simulink model "CAN_new"  (R2013b)
settings: Solver=FixedStepDiscrete  StartTime=0.0  StopTime=Inf  FixedStep=0.001  RelTol=1e-3
PostLoadFcn:
  | , if any(exist('dsrtsu_mdlpostloadfcn', 'file') == [2, 3, 6]), try dsrtsu_mdlpostloadfcn('Execute', bdroot); catch fprintf('Error in PostLoadFcn (dsrtsu_mdlpostloadfcn) for model "%s":\n %s\n', bdroot, lasterr); end, end,
undefined symbols (not defined in the file or in its folder): rticanmm_blockfcn, rticanmm_initfcn
libraries: rtimmsu_dsrtlib x4
(part 1 of 2)
settings Model: DSRTSU_INTERNAL_RTI_VER=440  DSRTSU_INTERNAL_RTI_TYPE=rti1401  RTICANMMDATA=struct('GeneralSetupData',struct('modelroot','C:\Users\Sebastian\Documents\GitHub\MA_Active_Steering_Dolly\DBC_Files','generalsettings',struct('filesettings',struct('destfolder',struct('Name','RTICANMM_FILES','Check',1),'buildfolder',struct('Name','.','Check',1),'AbsDestfolder',struct('Name','C:\Users\Sebastian\Documents\GitHub\MA_Active_Steering_Dolly\DBC_Files\RTICANMM_FILES'),'AbsBuildfolder',struct('Name','C:\Users\Sebastian\Documents\GitHub\MA_Active_Steering_Dolly\DBC_Files'))),'options',struct('addpaths',1,'rmpaths',1,'addtrcexclusion',logical(1),'cannavigator',struct('checkmonitoring',0),'show_usrtrc',0,'use_usrtrc',0,'addpath2usrmk',1),'advanced',struct('options',[1 1 1 1 1 1 1 1 1 1 1 1 1 1 1 1 1 1 1 1 1 1 1 1 1 1 1 1 1 1 1 1 1 1 1 1 1 1 1 1 1 1 1 1 1 1 1 1 1 1 1 1 1 1 1 1 1 1 1 1 1 1 1 1 1 1 1 1 1 1 1 1 1 1 1 1 1 1 1 1 1 1 1 1 1 1 1 1 1 1 1 1 1 1 1 1 1 1 1 1]),'MPSetup',{{}},'modelname','CAN_new','blockdata',struct('generalsettings',struct('filesettings',struct('destfolder',struct('Name','.','Check',1),'AbsDestfolder',struct('Name','T:\TOOL_SOURCES\CANnedy\m'),'buildfolder',struct('Name','.','Check',1),'AbsBuildfolder',struct('Name','C:\MATLAB6p5\work'))),'options',struct('addpaths',1,'rmpaths',1,'addpath2usrmk',1),'modelname','rticanmmlib','modelroot','T:\TOOL_SOURCES\CANnedy\m'),'MMType','RTICANMM','block',['CAN_new/Angle_Sensor/RTICANMM' char(10) 'GeneralSetup'],'RTI',struct('Type','RTI1401','Ver','7.2','Date','02-May-2014'),'version','3.0.735671.4434490741','userdata',struct('HostServiceChannelID',{{'Controller1','Controller2','Controller3'}})))  DSRTSU_INTERNAL_RTIFPGA=30  BufferReuse=off  Creator=Sebastian  LastModifiedBy=Sebastian
settings OptimizationCC: BlockReduction=off  OptimizeBlockIOStorage=off  BufferReuse=off  ExpressionFolding=off  LocalBlockOutputs=off
settings HardwareCC: ProdIntDivRoundTo=Zero  ProdEndianess=BigEndian  ProdHWDeviceType=Generic->Custom  TargetIntDivRoundTo=Zero  TargetEndianess=BigEndian  TargetHWDeviceType=Generic->Custom
settings RTWCC: SystemTargetFile=rti1401.tlc  MakeCommand=make_rti  TemplateMakefile=rti1401.tmf  Description=dSPACE DS1401 Hardware Platform  ProcessScript=rti1401_make_rtw_hook
settings STFCustomTargetCC: ParMdlRefBuildCompliant=on  GeneratePreprocessorConditionals=Disable all  SystemTargetFile=rti1401.tlc
settings GRTTargetCC: CompOptLevelCompliant=off  ConcurrentExecutionCompliant=off  CombineOutputUpdateFcns=off  MatFileLogging=off  GRTInterface=on  ExtModeMexFile=noextcomm

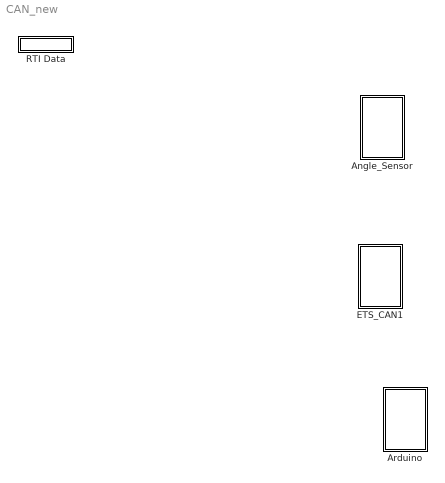
== system CAN_new ==
  Angle_Sensor : Subsystem
  Arduino : Subsystem
  ETS_CAN1 : Subsystem
  RTI Data : Subsystem  Tag=struct('RTIDataServer',struct('RTIDataServerVs','2','RTIModelDescription','struct(''main'',''CAN_new'',''sub'','''',''isMp'',0)'))  LoadFcn="if exist('rtidc'), try,  rtidc('DataHostBlockClbLoad', gcbh); catch, disp(['Warning: ''LoadFcn'' for RTI Data block failed: ' lasterr]); end, end,"  mask(RTI_DATA_HOST){}
      mask help:
      | RTI Data Block.
      | This block is used by RTI to store internal model-dependent data.
      | Please keep this block on the root level of the model. Deleting this block will result in data loss.
      |
      | NEVER DELETE OR COPY THIS BLOCK!
      settings: CopyFcn="if exist('rtidc'), try,  rtidc('DataHostBlockClbCopy', gcbh); catch, disp(['Warning: ''CopyFcn'' for RTI Data block failed: ' lasterr]); end, end,"  DeleteFcn="if exist('rtidc'), try,  rtidc('DataHostBlockClbDelete', gcbh); catch, disp(['Warning: ''DeleteFcn'' for RTI Data block failed: ' lasterr]); end, end,"  ModelCloseFcn="if exist('rtidc'), try,  rtidc('DataHostBlockClbModelClose', gcbh); catch, disp(['Warning: ''ModelCloseFcn'' for RTI Data block failed: ' lasterr]); end, end,"  PreSaveFcn="if exist('rtidc'), try,  rtidc('DataHostBlockClbPreSave', gcbh); catch, disp(['Warning: ''PreSaveFcn'' for RTI Data block failed: ' lasterr]); end, end,"  PostSaveFcn="if exist('rtidc'), try,  rtidc('DataHostBlockClbPostSave', gcbh); catch, disp(['Warning: ''PostSaveFcn'' for RTI Data block failed: ' lasterr]); end, end,"  NameChangeFcn="if exist('rtidc'), try,  rtidc('DataHostBlockClbNameChange', gcbh); catch, disp(['Warning: ''NameChangeFcn'' for RTI Data block failed: ' lasterr]); end, end,"
      mask Help:
      | RTI Data Block.
      | This block is used by RTI to store internal model-dependent data.
      | Please keep this block on the root level of the model. Deleting this block will result in data loss.
      | 
      | NEVER DELETE OR COPY THIS BLOCK!
      mask Display:
      | text(0.5, 0.5, 'RTI Data', 'HorizontalAlignment', 'center');
      | plot([1 0]);

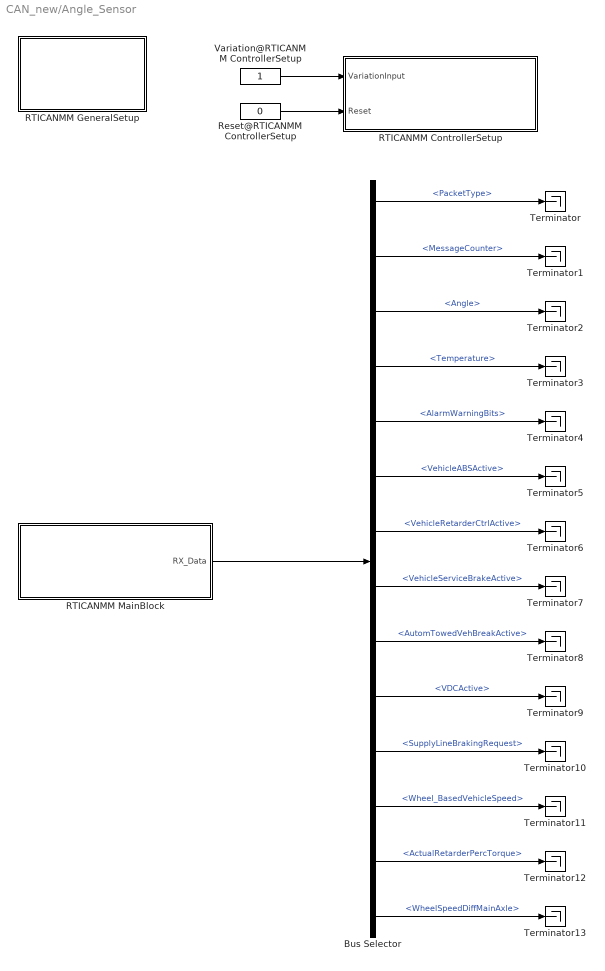
== system CAN_new/Angle_Sensor ==
  Bus Selector : BusSelector  OutputSignals=AngleSensor.PacketType,AngleSensor.MessageCounter,AngleSensor.Angle,AngleSensor.Temperature,AngleSensor.AlarmWarningBits,ISO11992_EBS21.VehicleABSActive,ISO11992_EBS21.VehicleRetarderCtrlActive,ISO11992_EBS21.VehicleServiceBrakeActive,ISO11992_EBS21.AutomTowedVehBreakActive,ISO11992_EBS21.VDCActive,ISO11992_EBS21.SupplyLineBrakingRequest,ISO11992_EBS21.Wheel_BasedVehicleSpeed,ISO11992_EBS21.ActualRetarderPercTorque,ISO11992_EBS21.WheelSpeedDiffMainAxle
  RTICANMM ControllerSetup : Subsystem  InitFcn=rticanmm_blockfcn('InitFcn', 'CANnedySetup', gcb)  ClipboardFcn=rticanmm_blockfcn('ClipboardFcn', 'CANnedySetup', gcb)  mask(RTICANMM){DSProperties=struct('RTI',struct('Version',uint32(1),'BlockType',struct('isSLSource',uint8(1),'isSLSink',uint8(1),'isHWSource',uint8(0),'isHWSink',uint8(0),'isSetup',uint8(0),'isInline',uint8(1),'isNonInline',uint8(0),'isInterrupt',uint8(0),'isChannelwise',uint8(0)),'IOBoardType','RTICANMM','UnitType','RTICANMM','Identifier','BUSSETUP','DialogType','SL','BlockSet','RTICANMM','SlaveProcessor','CAN')), CANMMProperties=struct('cannedy',struct('data',struct('options',struct('controllername','Controller1','controllernameautomatic',[],'loglevel','0','checkrealtime',0,'checkchangebaudrate',0,'sampletime','1.000','CANControllerStatus',0,'NumberofStuffErr',0,'NumberofFormErr',0,'NumberofAckErr',0,'NumberofBit0Err',0,'NumberofsuccrecRX',0,'Numberofsuccsent',0,'NumberofBit1Err',0,'NumberofCRCErr',0,'NumberoflostRX',0,'Busoff',0,'Busload',0,'OperationPending',0,'TxRetryCount',3,'addtrcexclusion',logical(1),'cannavigator',struct('checkmonitoring',0,'checkinternmonitoring',0),'show_usrtrc',0,'use_usrtrc',0),'modelroot','C:\Users\Sebastian\Desktop\DBC_Files','generalsettings',struct('setupdata',struct('board',['CAN Type 1'],'boardno',1,'channelno',1,'Type','STD','transceiver','ISO11898-2','busconfig','0x0','feedthrough','false','resistance',struct('r120',1,'roff',0,'r16',1,'r10',0),'baudrate','500','Frequency',[24 36],'samplemode',1,'commChannelTJA1041',6,'config',struct('standard',1,'advanced',0,'register',struct('btr0','0xC0','btr1','0x6F','sp','70','sjw','3','tseg1','15','tseg2','6','brp','0','smpl','0','btr0_36','0x41','btr1_36','0x1E','sp_36','88','sjw_36','1','tseg1_36','14','tseg2_36','1','brp_36','1','smpl_36','0','btr0_64','0x43','btr1_64','0x1C','sp_64','87','sjw_64','1','tseg1_64','12','tseg2_64','1','brp_64','3','smpl_64','0')),'channelcfg',struct('INTENDISABLE','CAN_INT_DISABLE','intenable',0),'SETUPID','RTICANMM_Controller1_ID','CONTROLLER_ID','CANMM_CTL_SETUP_Controller1','mainblock_includefile','RTICANMM_SETUP_Controller1','termination','TERMINATION_ON'),'filesettings',struct('destfolder',struct('Name','RTICANMM_FILES','Check',1),'buildfolder',struct('Name','.','Check',1))),'advanced',struct('options',[1 1 1 1 1 1 1 1 1 1 1 1 1 1 1 1 1 1 1 1 1 1 1 1 1 1 1 1 1 1 1 1 1 1 1 1 1 1 1 1 1 1 1 1 1 1 1 1 1 1 1 1 1 1 1 1 1 1 1 1 1 1 1 1 1 1 1 1 1 1 1 1 1 1 1 1 1 1 1 1 1 1 1 1 1 1 1 1 1 1 1 1 1 1 1 1 1 1 1 1]),'partialnetdata',struct('switchedon',0,'format','STD','idmask',['XXXXX XXXXXXXX XXXXXXXX XXXXXXXX'],'idcode','0','idfilter','0','datamaskused',0,'datalength','0','datamask','0x0000000000000000','partialnetworkenable',0)),'blk',['CAN_new/RTICANMM' char(10) 'ControllerSetup'],'allgeneratedfiles',{{'C:\Users\Sebastian\Desktop\DBC_Files\RTICANMM_FILES\RTICANMM_SETUP_Controller1.c','C:\Users\Sebastian\Desktop\DBC_Files\RTICANMM_FILES\RTICANMM_SETUP_Controller1.h','c:\users\sebastian\desktop\dbc_files\rticanmm_files\rticanmm_setup_controller1.mexw64'}},'ismp',logical(0),'BlockDataVersion','0.6.0','recreate',0),'CANnedynew',0,'CANnedySettings','Controller1','GeneratedFiles',{{'C:\Users\Sebastian\Desktop\DBC_Files\RTICANMM_FILES\RTICANMM_SETUP_Controller1.c','C:\Users\Sebastian\Desktop\DBC_Files\RTICANMM_FILES\RTICANMM_SETUP_Controller1.h','c:\users\sebastian\desktop\dbc_files\rticanmm_files\rticanmm_setup_controller1.mexw64'}},'SFCN','RTICANMM_SETUP_Controller1.c','HostService',struct('Tags',struct('DATA','RTICANMM_MonitorData','Enable','CANMMMonitor_Controller1','TimeStamp','MonitoringTimeStamp_Controller1'),'DATA',struct('Length',4),'Info',struct('Desc',{'ID','Service','Data1','Data2'}),'Names',struct('Enable','Monitoring_Enable','TimeStamp','Monitoring_TimeStamp'),'ChannelID',1)), CANMMType=CANnedySetup, CANMMFolder=C:\Users\Sebastian\Documents\GitHub\MA_Active_Steering_Dolly\DBC_Files, CANMMDestFolder=RTICANMM_FILES, CANMMSettings=Controller1, CANMMSFcn=RTICANMM_SETUP_Controller1, CANMMBoard=DS1401, CANMMBoardNum=1, CANMMChannel=1}
      settings: AttributesFormatString=%<CANMMSettings>: %<CANMMBoard>_B%<CANMMBoardNum>_C%<CANMMChannel>  CopyFcn=rticanmm_blockfcn('CopyFcn', 'CANnedySetup', gcb)  DeleteFcn=rticanmm_blockfcn('DeleteFcn', 'CANnedySetup', gcb)  ModelCloseFcn=rticanmm_blockfcn('ModelCloseFcn', 'CANnedySetup', gcb)  NameChangeFcn=rticanmm_blockfcn('NameChangeFcn', 'CANnedySetup', gcb)  OpenFcn=try, rticanmm_setup_gui('create',gcb); ; catch,errordlg({lasterr, '','Please check your RTI installation.'},['Error: ' upper(bdroot)], 'replace'); end  MoveFcn=rticanmm_blockfcn('MoveFcn', 'CANnedySetup', gcb)
      mask Help: eval('rticanmm_quickstart(''create'', gcb);', 'disp(lasterr);')
      mask Display:
      | disp('RTI CAN\nMultiMessage\nControllerSetup')
      | 
      | port_label('input', 1 , 'Variation')
      | port_label('input', 2 , 'Reset')
  RTICANMM GeneralSetup : Subsystem  InitFcn=rticanmm_initfcn(gcb, 'CANnedySettings')  ClipboardFcn=rticanmm_blockfcn('ClipboardFcn', 'CANnedySettings', gcb)  mask(RTICANMM){DSProperties=struct('RTI',struct('Version',uint32(1),'BlockType',struct('isSLSource',uint8(1),'isSLSink',uint8(1),'isHWSource',uint8(0),'isHWSink',uint8(0),'isSetup',uint8(0),'isInline',uint8(1),'isNonInline',uint8(0),'isInterrupt',uint8(0),'isChannelwise',uint8(0)),'IOBoardType','RTICANMM','UnitType','RTICANMM','Identifier','GENERALSETUP','DialogType','SL','BlockSet','RTICANMM','SlaveProcessor','CAN')), CANMMDestFolder=RTICANMM_FILES, CANMMBuildDir=., CANMMAddPaths=on, CANMMAddpathUserMake=on, CANMMRemovePathOnclose=on, CANMMType=CANnedySettings, CANMMProperties=struct('modelroot','C:\Users\Sebastian\Documents\GitHub\MA_Active_Steering_Dolly\DBC_Files','generalsettings',struct('filesettings',struct('destfolder',struct('Name','RTICANMM_FILES','Check',1),'buildfolder',struct('Name','.','Check',1),'AbsDestfolder',struct('Name','C:\Users\Sebastian\Documents\GitHub\MA_Active_Steering_Dolly\DBC_Files\RTICANMM_FILES'),'AbsBuildfolder',struct('Name','C:\Users\Sebastian\Documents\GitHub\MA_Active_Steering_Dolly\DBC_Files'))),'options',struct('addpaths',1,'rmpaths',1,'addtrcexclusion',logical(1),'cannavigator',struct('checkmonitoring',0),'show_usrtrc',0,'use_usrtrc',0,'addpath2usrmk',1),'advanced',struct('options',[1 1 1 1 1 1 1 1 1 1 1 1 1 1 1 1 1 1 1 1 1 1 1 1 1 1 1 1 1 1 1 1 1 1 1 1 1 1 1 1 1 1 1 1 1 1 1 1 1 1 1 1 1 1 1 1 1 1 1 1 1 1 1 1 1 1 1 1 1 1 1 1 1 1 1 1 1 1 1 1 1 1 1 1 1 1 1 1 1 1 1 1 1 1 1 1 1 1 1 1]),'MPSetup',{{}},'modelname','CAN_new','blockdata',struct('generalsettings',struct('filesettings',struct('destfolder',struct('Name','.','Check',1),'AbsDestfolder',struct('Name','T:\TOOL_SOURCES\CANnedy\m'),'buildfolder',struct('Name','.','Check',1),'AbsBuildfolder',struct('Name','C:\MATLAB6p5\work'))),'options',struct('addpaths',1,'rmpaths',1,'addpath2usrmk',1),'modelname','rticanmmlib','modelroot','T:\TOOL_SOURCES\CANnedy\m'),'MMType','RTICANMM','block',['CAN_new/Angle_Sensor/RTICANMM' char(10) 'GeneralSetup'],'RTI',struct('Type','RTI1401','Ver','7.2','Date','02-May-2014'),'version','3.0.735671.4434490741','userdata',struct('HostServiceChannelID',{{'Controller1','Controller2','Controller3'}}))}
      mask prompts: CANMMDestFolder "Destination Folder for generated Files:"; CANMMBuildDir "Build Directory (*_usr.mk, *_usr.trc)"; CANMMAddPaths "Add Paths automatically"; CANMMAddpathUserMake "Add Paths to UserMake-File"; CANMMRemovePathOnclose "Remove added Path on ModelClose"
      mask init:
      | rticanmm_initfcn(gcb,'CANnedyGeneralSettings')
      settings: CopyFcn=rticanmm_blockfcn('CopyFcn', 'CANnedySettings', gcb)  DeleteFcn=rticanmm_blockfcn('DeleteFcn', 'CANnedySettings', gcb)  ModelCloseFcn=rticanmm_blockfcn('CloseFcn', 'CANnedyGeneralSettings', gcb)  NameChangeFcn=rticanmm_blockfcn('NameChangeFcn', 'CANnedySettings', gcb)  OpenFcn=try, rticanmm_gs_gui('create',gcb), ; catch,errordlg({lasterr, '','Please check your RTI installation.'},['Error: ' upper(bdroot)], 'replace'); end  MoveFcn=rticanmm_blockfcn('MoveFcn', 'CANnedySettings', gcb)
      mask Help: eval('rticanmm_quickstart(''create'', gcb);', 'disp(lasterr);')
      mask Display: disp(sprintf(['RTI CAN\nMultiMessage\nGeneralSetup']))
  RTICANMM MainBlock : Subsystem  InitFcn=rticanmm_blockfcn('InitFcn', 'CANnedy', gcb)  ClipboardFcn=rticanmm_blockfcn('ClipboardFcn', 'CANnedy', gcb)  mask(RTICANMM){DSProperties=struct('RTI',struct('Version',uint32(1),'BlockType',struct('isSLSource',uint8(1),'isSLSink',uint8(1),'isHWSource',uint8(0),'isHWSink',uint8(0),'isSetup',uint8(0),'isInline',uint8(1),'isNonInline',uint8(0),'isInterrupt',uint8(0),'isChannelwise',uint8(0)),'IOBoardType','RTICANMM','UnitType','RTICANMM','Identifier','Mainblock','DialogType','SL','BlockSet','RTICANMM','SlaveProcessor','CAN')), CANMMProperties=struct('RTICANMMVersion','3.0','RTICANMMVersionIntern','3.0.735671.4434490741','RTICANMMDate','02-May-2014','Settings','RTICANMM_MAIN_CAN','UserTracePath','','ModelPath','C:\Users\Sebastian\Documents\GitHub\MA_Active_Steering_Dolly\DBC_Files','filesettings',struct('FileName','AngleSpeed.dbc','IsRelative',1,'ClusterId',1,'ClusterList',{{'default'}},'destfolder',struct('Name','RTICANMM_FILES','Check',1),'buildfolder',struct('Name','.','Check',1),'onlyfreerawcapture',0,'overlapping2variant',0),'onlyfreerawcapture',0,'Board',['CAN Type 1'],'BoardNum','1','ChannelNum','1','Variation','1','SetupId','Controller1','MARK',['7DBF185AE8E2AF6E949032F17CD527';'068CEB1B2D5027FC45531E1F7A9409';'09567626E24A705194943A5CB25188';'8B3CC76C9A9A67B6C72B37BE9D1636';'1A4B083466BA306CD50E4EA3714E2E'],'date','28-Jan-2015','clock',['28.01.2015 10:11:25'],'recreate',0,'RTIVER','RTI1401','j1939',0,'TRC',struct('include',1),'rtsupport',struct('XMLFile','C:\Users\Sebastian\Documents\GitHub\MA_Active_Steering_Dolly\DBC_Files\RTICANMM_FILES\RTICANMM_MAIN_CAN.xml','DBCXML',struct('Path','C:\Users\Sebastian\Documents\GitHub\MA_Active_Steering_Dolly\DBC_Files\RTICANMM_FILES\RTICANMM_MAIN_CAN_dbc.xml','support',1,'Name','AngleSpeed.dbc','Date',['11-Dez-2014 10:18:45'],'Type','extended','DBCSupport','ON'))), CANMMType=CANnedy, CANMMUserTraceMerged=off, CANMMUserTracePath=, CANMMChannelNum=1, CANMMBoardNum=1, CANMMDestFolder=RTICANMM_FILES, CANMMFolder=., CANMMSetupId=Controller1, CANMMsave2mat=['7DBF185AE8E2AF6E949032F17CD527';'068CEB1B2D5027FC45531E1F7A9409';'09567626E24A705194943A5CB25188';'8B3CC76C9A9A67B6C72B37BE9D1636';'1A4B083466BA306CD50E4EA3714E2E'], CANMMName=CAN, CANMMSettings=RTICANMM_MAIN_CAN, CANMMIntermediateTag=RTICANMM_MAIN_CAN_intermediate, CANMMsfcnname=RTICANMM_MAIN_CAN}
      mask init:
      | rticanmm_initfcn(gcb, CANMMType, CANMMsfcnname)
      settings: AttributesFormatString=Controller1[CAN]: DS1401_B1_C1_V1  CopyFcn=rticanmm_blockfcn('CopyFcn', 'CANnedy', gcb)  DeleteFcn=rticanmm_blockfcn('DeleteFcn', 'CANnedy', gcb)  ModelCloseFcn=rticanmm_blockfcn('ModelCloseFcn', 'CANnedy', gcb)  NameChangeFcn=rticanmm_blockfcn('NameChangeFcn', 'CANnedy', gcb)  OpenFcn=try, rticanmm_main_gui('create',gcb); ; catch,errordlg({lasterr, '','Please check your RTI installation.'},['Error: ' upper(bdroot)], 'replace'); end  MoveFcn=rticanmm_blockfcn('MoveFcn', 'CANnedy', gcb)
      mask Help: eval('rticanmm_quickstart(''create'', gcb);', 'disp(lasterr);')
      mask Display:
      | disp(sprintf('RTI CAN\nMultiMessage\nMainSetup'))
      | port_label('output', 1, 'RX Data')
  Reset@RTICANMM ControllerSetup : Constant  Value=0  OutDataTypeStr=boolean
  Terminator{,1..13} (14 alike) : Terminator
  Variation@RTICANMM ControllerSetup : Constant  OutDataTypeStr=uint8
  wires:
  RTICANMM MainBlock/1(RX_Data) -> Bus Selector/1
  Variation@RTICANMM ControllerSetup/1 -> RTICANMM ControllerSetup/1(VariationInput)
  Reset@RTICANMM ControllerSetup/1 -> RTICANMM ControllerSetup/2(Reset)
  Bus Selector/14 -> Terminator13/1  "<WheelSpeedDiffMainAxle>"
  Bus Selector/13 -> Terminator12/1  "<ActualRetarderPercTorque>"
  Bus Selector/12 -> Terminator11/1  "<Wheel_BasedVehicleSpeed>"
  Bus Selector/11 -> Terminator10/1  "<SupplyLineBrakingRequest>"
  Bus Selector/10 -> Terminator9/1  "<VDCActive>"
  Bus Selector/9 -> Terminator8/1  "<AutomTowedVehBreakActive>"
  Bus Selector/8 -> Terminator7/1  "<VehicleServiceBrakeActive>"
  Bus Selector/7 -> Terminator6/1  "<VehicleRetarderCtrlActive>"
  Bus Selector/6 -> Terminator5/1  "<VehicleABSActive>"
  Bus Selector/5 -> Terminator4/1  "<AlarmWarningBits>"
  Bus Selector/4 -> Terminator3/1  "<Temperature>"
  Bus Selector/3 -> Terminator2/1  "<Angle>"
  Bus Selector/2 -> Terminator1/1  "<MessageCounter>"
  Bus Selector/1 -> Terminator/1  "<PacketType>"

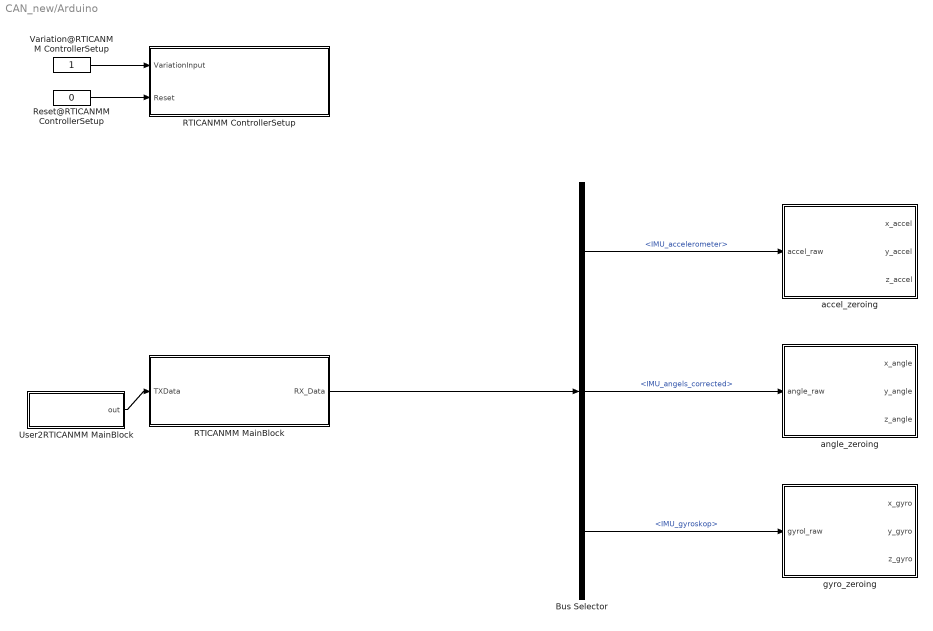
== system CAN_new/Arduino ==
  Bus Selector : BusSelector  OutputSignals=IMU_accelerometer,IMU_angels_corrected,IMU_gyroskop
  RTICANMM ControllerSetup : Subsystem  InitFcn=rticanmm_blockfcn('InitFcn', 'CANnedySetup', gcb)  ClipboardFcn=rticanmm_blockfcn('ClipboardFcn', 'CANnedySetup', gcb)  mask(RTICANMM){DSProperties=struct('RTI',struct('Version',uint32(1),'BlockType',struct('isSLSource',uint8(1),'isSLSink',uint8(1),'isHWSource',uint8(0),'isHWSink',uint8(0),'isSetup',uint8(0),'isInline',uint8(1),'isNonInline',uint8(0),'isInterrupt',uint8(0),'isChannelwise',uint8(0)),'IOBoardType','RTICANMM','UnitType','RTICANMM','Identifier','BUSSETUP','DialogType','SL','BlockSet','RTICANMM','SlaveProcessor','CAN')), CANMMProperties=struct('cannedy',struct('data',struct('options',struct('controllername','Controller3','controllernameautomatic',[],'loglevel','0','checkrealtime',0,'checkchangebaudrate',0,'sampletime','1.000','CANControllerStatus',0,'NumberofStuffErr',0,'NumberofFormErr',0,'NumberofAckErr',0,'NumberofBit0Err',0,'NumberofsuccrecRX',0,'Numberofsuccsent',0,'NumberofBit1Err',0,'NumberofCRCErr',0,'NumberoflostRX',0,'Busoff',0,'Busload',0,'OperationPending',0,'TxRetryCount',3,'addtrcexclusion',logical(1),'cannavigator',struct('checkmonitoring',0,'checkinternmonitoring',0),'show_usrtrc',0,'use_usrtrc',0),'modelroot','C:\Users\Sebastian\Documents\GitHub\MA_Active_Steering_Dolly\DBC_Files','generalsettings',struct('setupdata',struct('board',['CAN Type 1'],'boardno',2,'channelno',1,'Type','STD','transceiver','ISO11898-2','busconfig','0x0','feedthrough','false','resistance',struct('r120',1,'roff',0,'r16',1,'r10',0),'baudrate','500','Frequency',[24 36],'samplemode',1,'commChannelTJA1041',6,'config',struct('standard',1,'advanced',0,'register',struct('btr0','0xC0','btr1','0x6F','sp','70','sjw','3','tseg1','15','tseg2','6','brp','0','smpl','0','btr0_36','0x41','btr1_36','0x1E','sp_36','88','sjw_36','1','tseg1_36','14','tseg2_36','1','brp_36','1','smpl_36','0','btr0_64','0x43','btr1_64','0x1C','sp_64','87','sjw_64','1','tseg1_64','12','tseg2_64','1','brp_64','3','smpl_64','0')),'channelcfg',struct('INTENDISABLE','CAN_INT_DISABLE','intenable',0),'SETUPID','RTICANMM_Controller3_ID','CONTROLLER_ID','CANMM_CTL_SETUP_Controller3','mainblock_includefile','RTICANMM_SETUP_Controller3','termination','TERMINATION_ON'),'filesettings',struct('destfolder',struct('Name','RTICANMM_FILES','Check',1),'buildfolder',struct('Name','.','Check',1))),'advanced',struct('options',[1 1 1 1 1 1 1 1 1 1 1 1 1 1 1 1 1 1 1 1 1 1 1 1 1 1 1 1 1 1 1 1 1 1 1 1 1 1 1 1 1 1 1 1 1 1 1 1 1 1 1 1 1 1 1 1 1 1 1 1 1 1 1 1 1 1 1 1 1 1 1 1 1 1 1 1 1 1 1 1 1 1 1 1 1 1 1 1 1 1 1 1 1 1 1 1 1 1 1 1]),'partialnetdata',struct('switchedon',0,'format','STD','idmask',['XXXXX XXXXXXXX XXXXXXXX XXXXXXXX'],'idcode','0','idfilter','0','datamaskused',0,'datalength','0','datamask','0x0000000000000000','partialnetworkenable',0)),'blk',['CAN_new/Arduino/RTICANMM' char(10) 'ControllerSetup'],'allgeneratedfiles',{{'C:\Users\Sebastian\Documents\GitHub\MA_Active_Steering_Dolly\DBC_Files\RTICANMM_FILES\RTICANMM_SETUP_Controller3.c','C:\Users\Sebastian\Documents\GitHub\MA_Active_Steering_Dolly\DBC_Files\RTICANMM_FILES\RTICANMM_SETUP_Controller3.h','c:\users\sebastian\documents\github\ma_active_steering_dolly\dbc_files\rticanmm_files\rticanmm_setup_controller3.mexw64'}},'ismp',logical(0),'BlockDataVersion','0.6.0','recreate',0,'CANnedyTag','Controller3'),'CANnedynew',0,'CANnedySettings','Controller3','GeneratedFiles',{{'C:\Users\Sebastian\Documents\GitHub\MA_Active_Steering_Dolly\DBC_Files\RTICANMM_FILES\RTICANMM_SETUP_Controller3.c','C:\Users\Sebastian\Documents\GitHub\MA_Active_Steering_Dolly\DBC_Files\RTICANMM_FILES\RTICANMM_SETUP_Controller3.h','c:\users\sebastian\documents\github\ma_active_steering_dolly\dbc_files\rticanmm_files\rticanmm_setup_controller3.mexw64'}},'SFCN','RTICANMM_SETUP_Controller3.c','HostService',struct('Tags',struct('DATA','RTICANMM_MonitorData','Enable','CANMMMonitor_Controller3','TimeStamp','MonitoringTimeStamp_Controller3'),'DATA',struct('Length',4),'Info',struct('Desc',{'ID','Service','Data1','Data2'}),'Names',struct('Enable','Monitoring_Enable','TimeStamp','Monitoring_TimeStamp'),'ChannelID',3)), CANMMType=CANnedySetup, CANMMFolder=C:\Users\Sebastian\Documents\GitHub\MA_Active_Steering_Dolly\DBC_Files, CANMMDestFolder=RTICANMM_FILES, CANMMSettings=Controller3, CANMMSFcn=RTICANMM_SETUP_Controller3, CANMMBoard=DS1401, CANMMBoardNum=2, CANMMChannel=1}
      settings: AttributesFormatString=%<CANMMSettings>: %<CANMMBoard>_B%<CANMMBoardNum>_C%<CANMMChannel>  CopyFcn=rticanmm_blockfcn('CopyFcn', 'CANnedySetup', gcb)  DeleteFcn=rticanmm_blockfcn('DeleteFcn', 'CANnedySetup', gcb)  ModelCloseFcn=rticanmm_blockfcn('ModelCloseFcn', 'CANnedySetup', gcb)  NameChangeFcn=rticanmm_blockfcn('NameChangeFcn', 'CANnedySetup', gcb)  OpenFcn=try, rticanmm_setup_gui('create',gcb); ; catch,errordlg({lasterr, '','Please check your RTI installation.'},['Error: ' upper(bdroot)], 'replace'); end  MoveFcn=rticanmm_blockfcn('MoveFcn', 'CANnedySetup', gcb)
      mask Help: eval('rticanmm_quickstart(''create'', gcb);', 'disp(lasterr);')
      mask Display:
      | disp('RTI CAN\nMultiMessage\nControllerSetup')
      | 
      | port_label('input', 1 , 'Variation')
      | port_label('input', 2 , 'Reset')
  RTICANMM MainBlock : Subsystem  InitFcn=rticanmm_blockfcn('InitFcn', 'CANnedy', gcb)  ClipboardFcn=rticanmm_blockfcn('ClipboardFcn', 'CANnedy', gcb)  mask(RTICANMM){DSProperties=struct('RTI',struct('Version',uint32(1),'BlockType',struct('isSLSource',uint8(1),'isSLSink',uint8(1),'isHWSource',uint8(0),'isHWSink',uint8(0),'isSetup',uint8(0),'isInline',uint8(1),'isNonInline',uint8(0),'isInterrupt',uint8(0),'isChannelwise',uint8(0)),'IOBoardType','RTICANMM','UnitType','RTICANMM','Identifier','Mainblock','DialogType','SL','BlockSet','RTICANMM','SlaveProcessor','CAN')), CANMMProperties=struct('RTICANMMVersion','3.0','RTICANMMVersionIntern','3.0.735671.4434490741','RTICANMMDate','02-May-2014','Settings','RTICANMM_MAIN_CAN_Arduino','UserTracePath','','ModelPath','C:\Users\Sebastian\Documents\GitHub\MA_Active_Steering_Dolly\DBC_Files','filesettings',struct('FileName','can_drei_messages.dbc','IsRelative',1,'ClusterId',1,'ClusterList',{{'default'}},'destfolder',struct('Name','RTICANMM_FILES','Check',1),'buildfolder',struct('Name','.','Check',1),'onlyfreerawcapture',0,'overlapping2variant',0),'onlyfreerawcapture',0,'Board',['CAN Type 1'],'BoardNum','2','ChannelNum','1','Variation','1','SetupId','Controller3','MARK',['6BF6A98FD45F119C17313C933EB26D';'6E351746E33EAC9ACDAA678D4317E0';'0E214B6CBA412E4CCF79A36313B05A';'57BB44A8F5884E47BA0EE0078D0FCE';'AABE8D91A81494306A7D47DF46A86D'],'date','02-Feb-2015','clock',['02.02.2015 10:10:42'],'recreate',0,'RTIVER','RTI1401','j1939',0,'TRC',struct('include',1),'rtsupport',struct('XMLFile','C:\Users\Sebastian\Documents\GitHub\MA_Active_Steering_Dolly\DBC_Files\RTICANMM_FILES\RTICANMM_MAIN_CAN_Arduino.xml','DBCXML',struct('Path','C:\Users\Sebastian\Documents\GitHub\MA_Active_Steering_Dolly\DBC_Files\RTICANMM_FILES\RTICANMM_MAIN_CAN_Arduino_dbc.xml','support',1,'Name','can_drei_messages.dbc','Date',['28-Jan-2015 15:02:59'],'Type','standard','DBCSupport','ON'))), CANMMType=CANnedy, CANMMUserTraceMerged=off, CANMMUserTracePath=, CANMMChannelNum=1, CANMMBoardNum=2, CANMMDestFolder=RTICANMM_FILES, CANMMFolder=., CANMMSetupId=Controller3, CANMMsave2mat=['6BF6A98FD45F119C17313C933EB26D';'6E351746E33EAC9ACDAA678D4317E0';'0E214B6CBA412E4CCF79A36313B05A';'57BB44A8F5884E47BA0EE0078D0FCE';'AABE8D91A81494306A7D47DF46A86D'], CANMMName=CAN_Arduino, CANMMSettings=RTICANMM_MAIN_CAN_Arduino, CANMMIntermediateTag=RTICANMM_MAIN_CAN_Arduino_intermediate, CANMMsfcnname=RTICANMM_MAIN_CAN_Arduino}
      mask init:
      | rticanmm_initfcn(gcb, CANMMType, CANMMsfcnname)
      settings: AttributesFormatString=Controller3[CAN_Arduino]: DS1401_B2_C1_V1  CopyFcn=rticanmm_blockfcn('CopyFcn', 'CANnedy', gcb)  DeleteFcn=rticanmm_blockfcn('DeleteFcn', 'CANnedy', gcb)  ModelCloseFcn=rticanmm_blockfcn('ModelCloseFcn', 'CANnedy', gcb)  NameChangeFcn=rticanmm_blockfcn('NameChangeFcn', 'CANnedy', gcb)  OpenFcn=try, rticanmm_main_gui('create',gcb); ; catch,errordlg({lasterr, '','Please check your RTI installation.'},['Error: ' upper(bdroot)], 'replace'); end  MoveFcn=rticanmm_blockfcn('MoveFcn', 'CANnedy', gcb)
      mask Help: eval('rticanmm_quickstart(''create'', gcb);', 'disp(lasterr);')
      mask Display:
      | disp(sprintf('RTI CAN\nMultiMessage\nMainSetup'))
      | port_label('input', 1, 'TX Data')
      | port_label('output', 1, 'RX Data')
  Reset@RTICANMM ControllerSetup : Constant  Value=0  OutDataTypeStr=boolean
  User2RTICANMM MainBlock : Subsystem
      mask Display: disp('Mapping\nto RTICANMM')
  Variation@RTICANMM ControllerSetup : Constant  OutDataTypeStr=uint8
  accel_zeroing : Subsystem
  angle_zeroing : Subsystem
  gyro_zeroing : Subsystem
  wires:
  Reset@RTICANMM ControllerSetup/1 -> RTICANMM ControllerSetup/2(Reset)
  Variation@RTICANMM ControllerSetup/1 -> RTICANMM ControllerSetup/1(VariationInput)
  RTICANMM MainBlock/1(RX_Data) -> Bus Selector/1
  Bus Selector/2 -> angle_zeroing/1(angle_raw)  "<IMU_angels_corrected>"
  Bus Selector/3 -> gyro_zeroing/1(gyrol_raw)  "<IMU_gyroskop>"
  Bus Selector/1 -> accel_zeroing/1(accel_raw)  "<IMU_accelerometer>"
  User2RTICANMM MainBlock/1(out) -> RTICANMM MainBlock/1(TXData)

== system CAN_new/ETS_CAN1 ==
  Bus Selector : BusSelector  OutputSignals=AnalogInputVoltagesMessage1,AnalogInputVoltagesMessage2,CurrentMeasurementOutputs1,CurrentMeasurementOutputs2,DigitalInput,EtsDataMessage1,EtsDataMessage2,EtsDataMessage3,EtsDataMessage4,EtsDataMessage5,EtsSystemMessage,OilSupplyAssignmentMessage,OilSupplyRequestMessage,PowersupplyVoltageMessage1,PowersupplyVoltageMessage2,ResistanceMeasurementOutputs,SpeedMessage,StatusHighOutputPins,StatusLowOutputPins
  RTICANMM ControllerSetup : Subsystem  InitFcn=rticanmm_blockfcn('InitFcn', 'CANnedySetup', gcb)  ClipboardFcn=rticanmm_blockfcn('ClipboardFcn', 'CANnedySetup', gcb)  mask(RTICANMM){DSProperties=struct('RTI',struct('Version',uint32(1),'BlockType',struct('isSLSource',uint8(1),'isSLSink',uint8(1),'isHWSource',uint8(0),'isHWSink',uint8(0),'isSetup',uint8(0),'isInline',uint8(1),'isNonInline',uint8(0),'isInterrupt',uint8(0),'isChannelwise',uint8(0)),'IOBoardType','RTICANMM','UnitType','RTICANMM','Identifier','BUSSETUP','DialogType','SL','BlockSet','RTICANMM','SlaveProcessor','CAN')), CANMMProperties=struct('cannedy',struct('data',struct('options',struct('controllername','Controller2','controllernameautomatic',[],'loglevel','0','checkrealtime',0,'checkchangebaudrate',0,'sampletime','1.000','CANControllerStatus',0,'NumberofStuffErr',0,'NumberofFormErr',0,'NumberofAckErr',0,'NumberofBit0Err',0,'NumberofsuccrecRX',0,'Numberofsuccsent',0,'NumberofBit1Err',0,'NumberofCRCErr',0,'NumberoflostRX',0,'Busoff',0,'Busload',0,'OperationPending',0,'TxRetryCount',3,'addtrcexclusion',logical(1),'cannavigator',struct('checkmonitoring',0,'checkinternmonitoring',0),'show_usrtrc',0,'use_usrtrc',0),'modelroot','C:\Users\Sebastian\Desktop\DBC_Files','generalsettings',struct('setupdata',struct('board',['CAN Type 1'],'boardno',1,'channelno',2,'Type','STD','transceiver','ISO11898-2','busconfig','0x0','feedthrough','false','resistance',struct('r120',1,'roff',0,'r16',1,'r10',0),'baudrate','500','Frequency',[24 36],'samplemode',1,'commChannelTJA1041',6,'config',struct('standard',1,'advanced',0,'register',struct('btr0','0xC0','btr1','0x6F','sp','70','sjw','3','tseg1','15','tseg2','6','brp','0','smpl','0','btr0_36','0x41','btr1_36','0x1E','sp_36','88','sjw_36','1','tseg1_36','14','tseg2_36','1','brp_36','1','smpl_36','0','btr0_64','0x43','btr1_64','0x1C','sp_64','87','sjw_64','1','tseg1_64','12','tseg2_64','1','brp_64','3','smpl_64','0')),'channelcfg',struct('INTENDISABLE','CAN_INT_DISABLE','intenable',0),'SETUPID','RTICANMM_Controller2_ID','CONTROLLER_ID','CANMM_CTL_SETUP_Controller2','mainblock_includefile','RTICANMM_SETUP_Controller2','termination','TERMINATION_ON'),'filesettings',struct('destfolder',struct('Name','RTICANMM_FILES','Check',1),'buildfolder',struct('Name','.','Check',1))),'advanced',struct('options',[1 1 1 1 1 1 1 1 1 1 1 1 1 1 1 1 1 1 1 1 1 1 1 1 1 1 1 1 1 1 1 1 1 1 1 1 1 1 1 1 1 1 1 1 1 1 1 1 1 1 1 1 1 1 1 1 1 1 1 1 1 1 1 1 1 1 1 1 1 1 1 1 1 1 1 1 1 1 1 1 1 1 1 1 1 1 1 1 1 1 1 1 1 1 1 1 1 1 1 1]),'partialnetdata',struct('switchedon',0,'format','STD','idmask',['XXXXX XXXXXXXX XXXXXXXX XXXXXXXX'],'idcode','0','idfilter','0','datamaskused',0,'datalength','0','datamask','0x0000000000000000','partialnetworkenable',0)),'blk',['CAN_new/RTICANMM' char(10) 'ControllerSetup'],'allgeneratedfiles',{{'C:\Users\Sebastian\Desktop\DBC_Files\RTICANMM_FILES\RTICANMM_SETUP_Controller2.c','C:\Users\Sebastian\Desktop\DBC_Files\RTICANMM_FILES\RTICANMM_SETUP_Controller2.h','c:\users\sebastian\desktop\dbc_files\rticanmm_files\rticanmm_setup_controller2.mexw64'}},'ismp',logical(0),'BlockDataVersion','0.6.0','recreate',0),'CANnedynew',0,'CANnedySettings','Controller2','GeneratedFiles',{{'C:\Users\Sebastian\Desktop\DBC_Files\RTICANMM_FILES\RTICANMM_SETUP_Controller2.c','C:\Users\Sebastian\Desktop\DBC_Files\RTICANMM_FILES\RTICANMM_SETUP_Controller2.h','c:\users\sebastian\desktop\dbc_files\rticanmm_files\rticanmm_setup_controller2.mexw64'}},'SFCN','RTICANMM_SETUP_Controller2.c','HostService',struct('Tags',struct('DATA','RTICANMM_MonitorData','Enable','CANMMMonitor_Controller2','TimeStamp','MonitoringTimeStamp_Controller2'),'DATA',struct('Length',4),'Info',struct('Desc',{'ID','Service','Data1','Data2'}),'Names',struct('Enable','Monitoring_Enable','TimeStamp','Monitoring_TimeStamp'),'ChannelID',2)), CANMMType=CANnedySetup, CANMMFolder=C:\Users\Sebastian\Documents\GitHub\MA_Active_Steering_Dolly\DBC_Files, CANMMDestFolder=RTICANMM_FILES, CANMMSettings=Controller2, CANMMSFcn=RTICANMM_SETUP_Controller2, CANMMBoard=DS1401, CANMMBoardNum=1, CANMMChannel=2}
      settings: AttributesFormatString=%<CANMMSettings>: %<CANMMBoard>_B%<CANMMBoardNum>_C%<CANMMChannel>  CopyFcn=rticanmm_blockfcn('CopyFcn', 'CANnedySetup', gcb)  DeleteFcn=rticanmm_blockfcn('DeleteFcn', 'CANnedySetup', gcb)  ModelCloseFcn=rticanmm_blockfcn('ModelCloseFcn', 'CANnedySetup', gcb)  NameChangeFcn=rticanmm_blockfcn('NameChangeFcn', 'CANnedySetup', gcb)  OpenFcn=try, rticanmm_setup_gui('create',gcb); ; catch,errordlg({lasterr, '','Please check your RTI installation.'},['Error: ' upper(bdroot)], 'replace'); end  MoveFcn=rticanmm_blockfcn('MoveFcn', 'CANnedySetup', gcb)
      mask Help: eval('rticanmm_quickstart(''create'', gcb);', 'disp(lasterr);')
      mask Display:
      | disp('RTI CAN\nMultiMessage\nControllerSetup')
      | 
      | port_label('input', 1 , 'Variation')
      | port_label('input', 2 , 'Reset')
  RTICANMM MainBlock : Subsystem  InitFcn=rticanmm_blockfcn('InitFcn', 'CANnedy', gcb)  ClipboardFcn=rticanmm_blockfcn('ClipboardFcn', 'CANnedy', gcb)  mask(RTICANMM){DSProperties=struct('RTI',struct('Version',uint32(1),'BlockType',struct('isSLSource',uint8(1),'isSLSink',uint8(1),'isHWSource',uint8(0),'isHWSink',uint8(0),'isSetup',uint8(0),'isInline',uint8(1),'isNonInline',uint8(0),'isInterrupt',uint8(0),'isChannelwise',uint8(0)),'IOBoardType','RTICANMM','UnitType','RTICANMM','Identifier','Mainblock','DialogType','SL','BlockSet','RTICANMM','SlaveProcessor','CAN')), CANMMProperties=struct('RTICANMMVersion','3.0','RTICANMMVersionIntern','3.0.735671.4434490741','RTICANMMDate','02-May-2014','Settings','RTICANMM_MAIN_CAN_2','UserTracePath','','ModelPath','C:\Users\Sebastian\Documents\GitHub\MA_Active_Steering_Dolly\DBC_Files','filesettings',struct('FileName','0_ETS_CAN1.dbc','IsRelative',1,'ClusterId',1,'ClusterList',{{'default'}},'destfolder',struct('Name','RTICANMM_FILES','Check',1),'buildfolder',struct('Name','.','Check',1),'onlyfreerawcapture',0,'overlapping2variant',0),'onlyfreerawcapture',0,'Board',['CAN Type 1'],'BoardNum','1','ChannelNum','2','Variation','1','SetupId','Controller2','MARK',['7E2C310E5D7A02EAAC5A3BF2543FC9';'3CDC773D0500695099811511701E62';'7FDBC04255674F76D27161330D00F8';'1B983A09301517E09D3C133D24A7BA';'680B881186EB29AD0894DAC3AB5E07'],'date','30-Jan-2015','clock',['30.01.2015 11:52:31'],'recreate',0,'RTIVER','RTI1401','j1939',1,'TRC',struct('include',1),'rtsupport',struct('XMLFile','C:\Users\Sebastian\Documents\GitHub\MA_Active_Steering_Dolly\DBC_Files\RTICANMM_FILES\RTICANMM_MAIN_CAN_2.xml','DBCXML',struct('Path','C:\Users\Sebastian\Documents\GitHub\MA_Active_Steering_Dolly\DBC_Files\RTICANMM_FILES\RTICANMM_MAIN_CAN_2_dbc.xml','support',1,'Name','0_ETS_CAN1.dbc','Date',['11-Dez-2014 10:18:52'],'Type','J1939','DBCSupport','ON'))), CANMMType=CANnedy, CANMMUserTraceMerged=off, CANMMUserTracePath=, CANMMChannelNum=2, CANMMBoardNum=1, CANMMDestFolder=RTICANMM_FILES, CANMMFolder=., CANMMSetupId=Controller2, CANMMsave2mat=['7E2C310E5D7A02EAAC5A3BF2543FC9';'3CDC773D0500695099811511701E62';'7FDBC04255674F76D27161330D00F8';'1B983A09301517E09D3C133D24A7BA';'680B881186EB29AD0894DAC3AB5E07'], CANMMName=CAN_2, CANMMSettings=RTICANMM_MAIN_CAN_2, CANMMIntermediateTag=RTICANMM_MAIN_CAN_2_intermediate, CANMMsfcnname=RTICANMM_MAIN_CAN_2}
      mask init:
      | rticanmm_initfcn(gcb, CANMMType, CANMMsfcnname)
      settings: AttributesFormatString=Controller2[CAN_2]: DS1401_B1_C2_V1  CopyFcn=rticanmm_blockfcn('CopyFcn', 'CANnedy', gcb)  DeleteFcn=rticanmm_blockfcn('DeleteFcn', 'CANnedy', gcb)  ModelCloseFcn=rticanmm_blockfcn('ModelCloseFcn', 'CANnedy', gcb)  NameChangeFcn=rticanmm_blockfcn('NameChangeFcn', 'CANnedy', gcb)  OpenFcn=try, rticanmm_main_gui('create',gcb); ; catch,errordlg({lasterr, '','Please check your RTI installation.'},['Error: ' upper(bdroot)], 'replace'); end  MoveFcn=rticanmm_blockfcn('MoveFcn', 'CANnedy', gcb)
      mask Help: eval('rticanmm_quickstart(''create'', gcb);', 'disp(lasterr);')
      mask Display:
      | disp(sprintf('RTI CAN\nMultiMessage\nMainSetup'))
      | port_label('output', 1, 'RX Data')
  Reset@RTICANMM ControllerSetup : Constant  Value=0  OutDataTypeStr=boolean
  Variation@RTICANMM ControllerSetup : Constant  OutDataTypeStr=uint8
  wires:
  Reset@RTICANMM ControllerSetup/1 -> RTICANMM ControllerSetup/2(Reset)
  Variation@RTICANMM ControllerSetup/1 -> RTICANMM ControllerSetup/1(VariationInput)
  RTICANMM MainBlock/1(RX_Data) -> Bus Selector/1

== system CAN_new/RTI Data ==
  RTI Data Store : Subsystem  Tag="struct('public',struct('sub',struct('name',{{'CAN_new'}},'data',{{struct('TH',struct('thTaskInfo',struct('taskType',{'TIMER','HWINT','TMRINT','SWINT','GLINT'},'tasksNumOf',{1,0,0,0,0},'srcIds',{{'TIMERA'},{},{},{},{}},'taskNames',{{['Timer Task 1']},{},{},{},{}})),'th_tc',struct('dataType','TASK','taskGroupId','','taskGroupList',{{}},'taskSchedulingPolicy','FCFS','taskType','TIMER','blkh',-1,'srcId','TIMERA','srcSgnName',['Timer A interrupt'],'srcCpuName','','taskName',['Timer Task 1  [0.001] s'],'taskNameDisplayExt','','smplTime',0.001,'smplTimeOffs',0,'hasFixedPriority',0,'priority',1,'hasFixedOvc',0,'ovcType',1,'ovcMax',1),'tc_th',struct('dataType','TASK','taskGroupId','','taskGroupList',{{}},'taskSchedulingPolicy','FCFS','taskType','TIMER','blkh',-1,'srcId','TIMERA','srcSgnName',['Timer A interrupt'],'srcCpuName','','taskName',['Timer Task 1  [0.001] s'],'taskNameDisplayExt','','smplTime',0.001,'smplTimeOffs',0,'hasFixedPriority',0,'priority',1,'hasFixedOvc',0,'ovcType',1,'ovcMax',1))}})),'private',struct('version',struct('dsVer',uint32(2)),'access',struct('modified',['02-Feb-2015 10:54:09'],'type','Model','isPerm',1)))"  mask(RTI_DATA_STORE){}
      mask help:
      | RTI Data Store Block. This block is used by RTI to store internal model dependent data. Deleting this block will result in data loss.
      |
      | NEVER DELETE, COPY, OR MODIFY THIS BLOCK!
      mask Help:
      | RTI Data Store Block. This block is used by RTI to store internal model dependent data. Deleting this block will result in data loss.
      | 
      | NEVER DELETE, COPY, OR MODIFY THIS BLOCK!
      mask Display: text(0.5, 0.5, ' ', 'HorizontalAlignment', 'center');

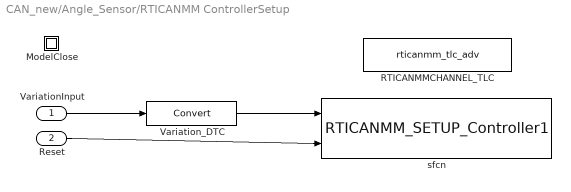
== system CAN_new/Angle_Sensor/RTICANMM ControllerSetup ==
  VariationInput : Inport
  Reset : Inport  Port=2
  ModelClose : Subsystem  mask(RTICANMMModelClose){}
  RTICANMMCHANNEL_TLC : S-Function  FunctionName=rticanmm_tlc_adv  Parameters=1401,1,1,0,500,'unused'  EnableBusSupport=off  mask(RTICANMMCHANNEL_TLC){}
  Variation_DTC : DataTypeConversion  SaturateOnIntegerOverflow=on  RndMeth=Zero
  sfcn : S-Function  InitFcn=rticanmm_initfcn(gcb, 'SFCNs')  FunctionName=RTICANMM_SETUP_Controller1  EnableBusSupport=off
      mask init:
      | rticanmm_initfcn(gcb, 'SFCNs')
  wires:
  Reset/1 -> sfcn/2
  VariationInput/1 -> Variation_DTC/1
  Variation_DTC/1 -> sfcn/1

== system CAN_new/Angle_Sensor/RTICANMM GeneralSetup ==
  Constant : Constant
  ModelClose : Subsystem  mask(RTICANMMModelClose){}
  TRC Exclusion : rtimmsu_dsrtlib/TRC Exclusion
  Terminator : Terminator
  wires:
  Constant/1 -> Terminator/1

== system CAN_new/Angle_Sensor/RTICANMM MainBlock ==
  ModelClose : Subsystem  mask(RTICANMMModelClose){}
  TRC Exclusion : rtimmsu_dsrtlib/TRC Exclusion
  converter : Subsystem  mask(CANnedyVector2Bus){}
      mask help: Do not change.
      mask Display: disp('Vector to\nBus')
  sfcn : S-Function  InitFcn=rticanmm_initfcn(gcb, 'SFCNs')  FunctionName=RTICANMM_MAIN_CAN  EnableBusSupport=off
      mask init:
      | rticanmm_initfcn(gcb, 'SFCNs')
  RX_Data : Outport
  wires:
  converter/1(out) -> RX_Data/1
  sfcn/1 -> converter/1(in_1)
  sfcn/2 -> converter/2(in_2)
  sfcn/3 -> converter/3(in_3)
  sfcn/4 -> converter/4(in_4)
  sfcn/5 -> converter/5(in_5)
  sfcn/6 -> converter/6(in_6)
  sfcn/7 -> converter/7(in_7)
  sfcn/8 -> converter/8(in_8)
  sfcn/9 -> converter/9(in_9)
  sfcn/10 -> converter/10(in_10)
  sfcn/11 -> converter/11(in_11)
  sfcn/12 -> converter/12(in_12)
  sfcn/13 -> converter/13(in_13)
  sfcn/14 -> converter/14(in_14)

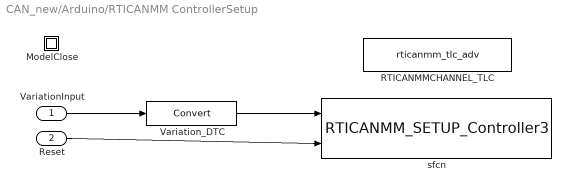
== system CAN_new/Arduino/RTICANMM ControllerSetup ==
  VariationInput : Inport
  Reset : Inport  Port=2
  ModelClose : Subsystem  mask(RTICANMMModelClose){}
  RTICANMMCHANNEL_TLC : S-Function  FunctionName=rticanmm_tlc_adv  Parameters=1401,2,1,0,500,'unused'  EnableBusSupport=off  mask(RTICANMMCHANNEL_TLC){}
  Variation_DTC : DataTypeConversion  SaturateOnIntegerOverflow=on  RndMeth=Zero
  sfcn : S-Function  InitFcn=rticanmm_initfcn(gcb, 'SFCNs')  FunctionName=RTICANMM_SETUP_Controller3  EnableBusSupport=off
      mask init:
      | rticanmm_initfcn(gcb, 'SFCNs')
  wires:
  Reset/1 -> sfcn/2
  VariationInput/1 -> Variation_DTC/1
  Variation_DTC/1 -> sfcn/1

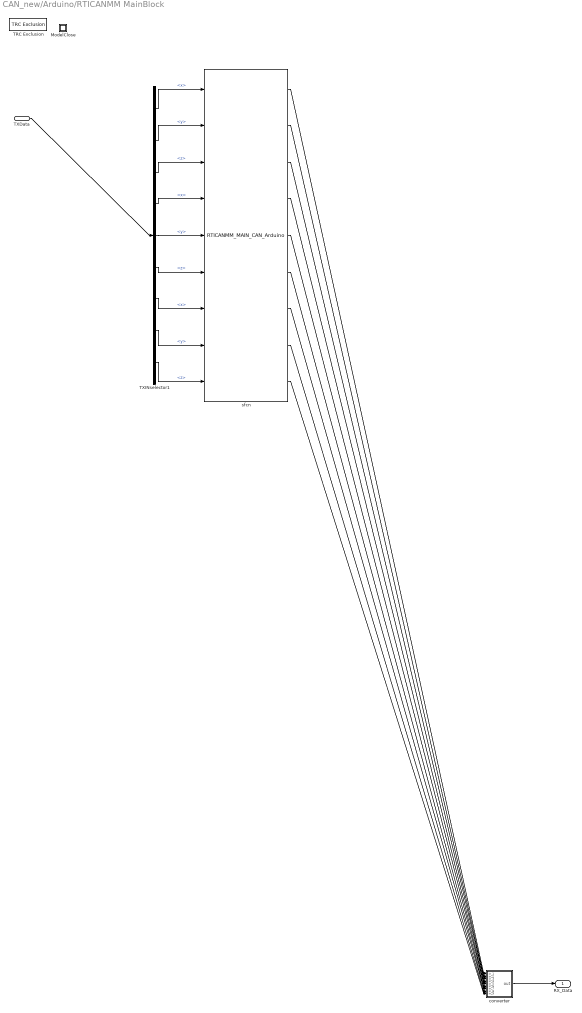
== system CAN_new/Arduino/RTICANMM MainBlock ==
  TXData : Inport
  ModelClose : Subsystem  mask(RTICANMMModelClose){}
  TRC Exclusion : rtimmsu_dsrtlib/TRC Exclusion
  TXINselector1 : BusSelector  OutputSignals=IMU_accelerometer.x,IMU_accelerometer.y,IMU_accelerometer.z,IMU_angels_corrected.x,IMU_angels_corrected.y,IMU_angels_corrected.z,IMU_gyroskop.x,IMU_gyroskop.y,IMU_gyroskop.z
  converter : Subsystem  mask(CANnedyVector2Bus){}
      mask help: Do not change.
      mask Display: disp('Vector to\nBus')
  sfcn : S-Function  InitFcn=rticanmm_initfcn(gcb, 'SFCNs')  FunctionName=RTICANMM_MAIN_CAN_Arduino  EnableBusSupport=off
      mask init:
      | rticanmm_initfcn(gcb, 'SFCNs')
  RX_Data : Outport
  wires:
  TXData/1 -> TXINselector1/1
  TXINselector1/1 -> sfcn/1  "<x>"
  TXINselector1/2 -> sfcn/2  "<y>"
  TXINselector1/3 -> sfcn/3  "<z>"
  TXINselector1/4 -> sfcn/4  "<x>"
  TXINselector1/5 -> sfcn/5  "<y>"
  TXINselector1/6 -> sfcn/6  "<z>"
  TXINselector1/7 -> sfcn/7  "<x>"
  TXINselector1/8 -> sfcn/8  "<y>"
  TXINselector1/9 -> sfcn/9  "<z>"
  converter/1(out) -> RX_Data/1
  sfcn/1 -> converter/1(in_1)
  sfcn/2 -> converter/2(in_2)
  sfcn/3 -> converter/3(in_3)
  sfcn/4 -> converter/4(in_4)
  sfcn/5 -> converter/5(in_5)
  sfcn/6 -> converter/6(in_6)
  sfcn/7 -> converter/7(in_7)
  sfcn/8 -> converter/8(in_8)
  sfcn/9 -> converter/9(in_9)

== system CAN_new/Arduino/User2RTICANMM MainBlock ==
  IMU_accelerometer : Subsystem
  IMU_angels_corrected : Subsystem
  IMU_gyroskop : Subsystem
  buscreator : BusCreator  Inputs=3
  out : Outport
  wires:
  IMU_accelerometer/1(out) -> buscreator/1  "IMU_accelerometer"
  IMU_angels_corrected/1(out) -> buscreator/2  "IMU_angels_corrected"
  IMU_gyroskop/1(out) -> buscreator/3  "IMU_gyroskop"
  buscreator/1 -> out/1  "CAN"

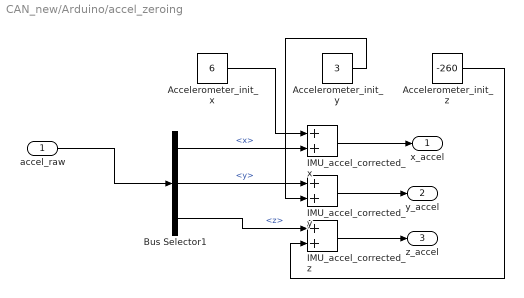
== system CAN_new/Arduino/accel_zeroing ==
  accel_raw : Inport
  Accelerometer_init_x : Constant  Value=6
  Accelerometer_init_y : Constant  Value=3
  "Accelerometer_init_z " : Constant  Value=-260
  Bus Selector1 : BusSelector  OutputSignals=x,y,z
  IMU_accel_corrected_x : Sum
  IMU_accel_corrected_y : Sum
  IMU_accel_corrected_z : Sum
  x_accel : Outport
  "y_accel " : Outport  Port=2
  z_accel : Outport  Port=3
  wires:
  accel_raw/1 -> Bus Selector1/1
  Accelerometer_init_x/1 -> IMU_accel_corrected_x/1
  Bus Selector1/2 -> IMU_accel_corrected_y/1  "<y>"
  Bus Selector1/1 -> IMU_accel_corrected_x/2  "<x>"
  Accelerometer_init_y/1 -> IMU_accel_corrected_y/2
  Bus Selector1/3 -> IMU_accel_corrected_z/1  "<z>"
  IMU_accel_corrected_x/1 -> x_accel/1
  "Accelerometer_init_z "/1 -> IMU_accel_corrected_z/2
  IMU_accel_corrected_y/1 -> "y_accel "/1
  IMU_accel_corrected_z/1 -> z_accel/1

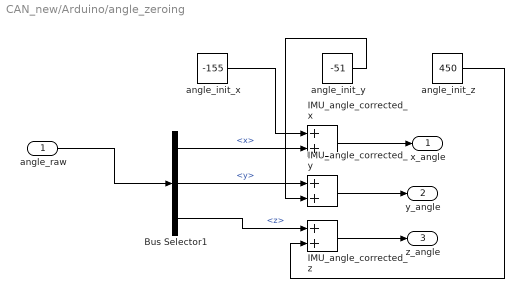
== system CAN_new/Arduino/angle_zeroing ==
  angle_raw : Inport
  Bus Selector1 : BusSelector  OutputSignals=x,y,z
  IMU_angle_corrected_x : Sum
  IMU_angle_corrected_y : Sum
  IMU_angle_corrected_z : Sum
  angle_init_x : Constant  Value=-155
  angle_init_y : Constant  Value=-51
  "angle_init_z " : Constant  Value=450
  x_angle : Outport
  y_angle : Outport  Port=2
  z_angle : Outport  Port=3
  wires:
  angle_raw/1 -> Bus Selector1/1
  angle_init_x/1 -> IMU_angle_corrected_x/1
  Bus Selector1/2 -> IMU_angle_corrected_y/1  "<y>"
  Bus Selector1/1 -> IMU_angle_corrected_x/2  "<x>"
  angle_init_y/1 -> IMU_angle_corrected_y/2
  Bus Selector1/3 -> IMU_angle_corrected_z/1  "<z>"
  IMU_angle_corrected_x/1 -> x_angle/1
  "angle_init_z "/1 -> IMU_angle_corrected_z/2
  IMU_angle_corrected_y/1 -> y_angle/1
  IMU_angle_corrected_z/1 -> z_angle/1

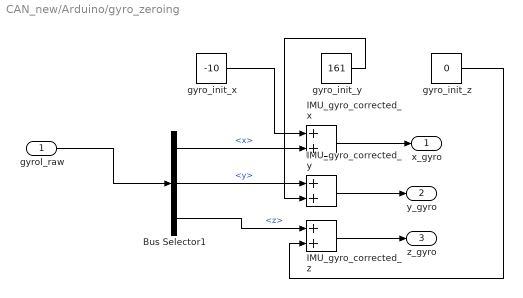
== system CAN_new/Arduino/gyro_zeroing ==
  gyrol_raw : Inport
  Bus Selector1 : BusSelector  OutputSignals=x,y,z
  IMU_gyro_corrected_x : Sum
  IMU_gyro_corrected_y : Sum
  IMU_gyro_corrected_z : Sum
  gyro_init_x : Constant  Value=-10
  gyro_init_y : Constant  Value=161
  "gyro_init_z " : Constant  Value=0
  x_gyro : Outport
  y_gyro : Outport  Port=2
  z_gyro : Outport  Port=3
  wires:
  gyrol_raw/1 -> Bus Selector1/1
  gyro_init_x/1 -> IMU_gyro_corrected_x/1
  Bus Selector1/2 -> IMU_gyro_corrected_y/1  "<y>"
  Bus Selector1/1 -> IMU_gyro_corrected_x/2  "<x>"
  gyro_init_y/1 -> IMU_gyro_corrected_y/2
  Bus Selector1/3 -> IMU_gyro_corrected_z/1  "<z>"
  IMU_gyro_corrected_x/1 -> x_gyro/1
  "gyro_init_z "/1 -> IMU_gyro_corrected_z/2
  IMU_gyro_corrected_y/1 -> y_gyro/1
  IMU_gyro_corrected_z/1 -> z_gyro/1

== system CAN_new/ETS_CAN1/RTICANMM ControllerSetup ==
  VariationInput : Inport
  Reset : Inport  Port=2
  ModelClose : Subsystem  mask(RTICANMMModelClose){}
  RTICANMMCHANNEL_TLC : S-Function  FunctionName=rticanmm_tlc_adv  Parameters=1401,1,2,0,500,'unused'  EnableBusSupport=off  mask(RTICANMMCHANNEL_TLC){}
  Variation_DTC : DataTypeConversion  SaturateOnIntegerOverflow=on  RndMeth=Zero
  sfcn : S-Function  InitFcn=rticanmm_initfcn(gcb, 'SFCNs')  FunctionName=RTICANMM_SETUP_Controller2  EnableBusSupport=off
      mask init:
      | rticanmm_initfcn(gcb, 'SFCNs')
  wires:
  Reset/1 -> sfcn/2
  VariationInput/1 -> Variation_DTC/1
  Variation_DTC/1 -> sfcn/1

== system CAN_new/ETS_CAN1/RTICANMM MainBlock ==
  ModelClose : Subsystem  mask(RTICANMMModelClose){}
  TRC Exclusion : rtimmsu_dsrtlib/TRC Exclusion
  converter : Subsystem  mask(CANnedyVector2Bus){}
      mask help: Do not change.
      mask Display: disp('Vector to\nBus')
  sfcn : S-Function  InitFcn=rticanmm_initfcn(gcb, 'SFCNs')  FunctionName=RTICANMM_MAIN_CAN_2  EnableBusSupport=off
      mask init:
      | rticanmm_initfcn(gcb, 'SFCNs')
  RX_Data : Outport
  wires:
  converter/1(out) -> RX_Data/1
  sfcn/1 -> converter/1(in_1)
  sfcn/2 -> converter/2(in_2)
  sfcn/3 -> converter/3(in_3)
  sfcn/4 -> converter/4(in_4)
  sfcn/5 -> converter/5(in_5)
  sfcn/6 -> converter/6(in_6)
  sfcn/7 -> converter/7(in_7)
  sfcn/8 -> converter/8(in_8)
  sfcn/9 -> converter/9(in_9)
  sfcn/10 -> converter/10(in_10)
  sfcn/11 -> converter/11(in_11)
  sfcn/12 -> converter/12(in_12)
  sfcn/13 -> converter/13(in_13)
  sfcn/14 -> converter/14(in_14)
  sfcn/15 -> converter/15(in_15)
  sfcn/16 -> converter/16(in_16)
  sfcn/17 -> converter/17(in_17)
  sfcn/18 -> converter/18(in_18)
  sfcn/19 -> converter/19(in_19)
  sfcn/20 -> converter/20(in_20)
  sfcn/21 -> converter/21(in_21)
  sfcn/22 -> converter/22(in_22)
  sfcn/23 -> converter/23(in_23)
  sfcn/24 -> converter/24(in_24)
  sfcn/25 -> converter/25(in_25)
  sfcn/26 -> converter/26(in_26)
  sfcn/27 -> converter/27(in_27)
  sfcn/28 -> converter/28(in_28)
  sfcn/29 -> converter/29(in_29)
  sfcn/30 -> converter/30(in_30)
  sfcn/31 -> converter/31(in_31)
  sfcn/32 -> converter/32(in_32)
  sfcn/33 -> converter/33(in_33)
  sfcn/34 -> converter/34(in_34)
  sfcn/35 -> converter/35(in_35)
  sfcn/36 -> converter/36(in_36)
  sfcn/37 -> converter/37(in_37)
  sfcn/38 -> converter/38(in_38)
  sfcn/39 -> converter/39(in_39)
  sfcn/40 -> converter/40(in_40)
  sfcn/41 -> converter/41(in_41)
  sfcn/42 -> converter/42(in_42)
  sfcn/43 -> converter/43(in_43)
  sfcn/44 -> converter/44(in_44)
  sfcn/45 -> converter/45(in_45)
  sfcn/46 -> converter/46(in_46)
  sfcn/47 -> converter/47(in_47)
  sfcn/48 -> converter/48(in_48)
  sfcn/49 -> converter/49(in_49)
  sfcn/50 -> converter/50(in_50)
  sfcn/51 -> converter/51(in_51)
  sfcn/52 -> converter/52(in_52)
  sfcn/53 -> converter/53(in_53)
  sfcn/54 -> converter/54(in_54)
  sfcn/55 -> converter/55(in_55)
  sfcn/56 -> converter/56(in_56)
  sfcn/57 -> converter/57(in_57)
  sfcn/58 -> converter/58(in_58)
  sfcn/59 -> converter/59(in_59)
  sfcn/60 -> converter/60(in_60)
  sfcn/61 -> converter/61(in_61)
  sfcn/62 -> converter/62(in_62)
  sfcn/63 -> converter/63(in_63)
  sfcn/64 -> converter/64(in_64)
  sfcn/65 -> converter/65(in_65)
  sfcn/66 -> converter/66(in_66)
  sfcn/67 -> converter/67(in_67)
  sfcn/68 -> converter/68(in_68)
  sfcn/69 -> converter/69(in_69)
  sfcn/70 -> converter/70(in_70)
  sfcn/71 -> converter/71(in_71)
  sfcn/72 -> converter/72(in_72)
  sfcn/73 -> converter/73(in_73)
  sfcn/74 -> converter/74(in_74)
  sfcn/75 -> converter/75(in_75)
  sfcn/76 -> converter/76(in_76)
  sfcn/77 -> converter/77(in_77)
  sfcn/78 -> converter/78(in_78)
  sfcn/79 -> converter/79(in_79)
  sfcn/80 -> converter/80(in_80)
  sfcn/81 -> converter/81(in_81)
  sfcn/82 -> converter/82(in_82)
  sfcn/83 -> converter/83(in_83)
  sfcn/84 -> converter/84(in_84)
  sfcn/85 -> converter/85(in_85)
  sfcn/86 -> converter/86(in_86)
  sfcn/87 -> converter/87(in_87)
  sfcn/88 -> converter/88(in_88)
  sfcn/89 -> converter/89(in_89)
  sfcn/90 -> converter/90(in_90)
  sfcn/91 -> converter/91(in_91)
  sfcn/92 -> converter/92(in_92)
  sfcn/93 -> converter/93(in_93)
  sfcn/94 -> converter/94(in_94)
  sfcn/95 -> converter/95(in_95)
  sfcn/96 -> converter/96(in_96)
  sfcn/97 -> converter/97(in_97)
